simulink model "F16ASYM_Controlled_AoA"  (R2012b)
settings: Solver=ode3  SolverMode=SingleTasking  StartTime=0.0  StopTime=inf  FixedStep=T_sim  RelTol=1e-3
InitFcn:
  | load('NN_c_weights_Last_stable.mat')
values from neighbouring files (symbols this model uses):
  K_b_AoA = params(3)    [Cost_function.m]
  K_b_q = params(4)    [Cost_function.m]
  learning = 20    [Scheduling_desing.m]
  Model_used_flag = 1    [Scheduling_desing.m]
  reg_param = 0.5    [Scheduling_desing.m]
  T_sim = 0.02    [Scheduling_desing.m]
  tau_AoA = params(1)    [Cost_function.m]
  tau_q = params(2)    [Cost_function.m]
  Theta_1_roll_last = [0.00183613313267 0.00115998993235 0.0006676025148 0.00194921904952 0.00134963559861 0.00034352059664 0.000447169388141 0.00146749660935 0.00110199952389 7.77922383894e-05 0.00109492833348 0.00192687590535 ... (360 elements, 30x12)]    [NN_i_weights_LAST_STABLE.mat]
  Theta_2_roll_last = [0.000469743069697 0.000355923851088 0.00180035760697 0.00191855117771 0.00118851504447 0.0013331642065 0.0013164316578 0.000643981263341 0.00176817665434 0.000113802099363 0.000426534542462 0.00113815782354 ... (620 elements, 20x31)]    [NN_i_weights_LAST_STABLE.mat]
  Theta_3_roll_last = [9.62071520568e-05 -0.000389870886846 2.08260845013e-05 0.000140787743673 -0.000917525755397 -0.0014324207578 -0.00154701573815 -0.00131544476264 -0.00101205584381 5.06515794689e-05 -0.00111443483676 -0.00143957416141 ... (21 elements, 1x21)]    [NN_i_weights_LAST_STABLE.mat]
  V_long_lastA_w_z = [0.352826086601 -0.253633004548 -0.642535042878 0.237749930435 -0.618390629538 0.858074761295 0.268211230628 -0.448715080196 -0.0406384631192 0.401147605577 0.60598427709 0.0500551915851 ... (300 elements, 30x10)]    [NN_i_weights_LAST_STABLE.mat]
  V_long_lastAoA = [0.0774300162379 0.0911421319631 0.0352371192557 0.0542170286952 0.0651171200844 0.0177112012707 0.0982957728448 0.000259994642558 0.0194724569123 0.0466321328252 0.0556687953852 0.0252668067142 ... (300 elements, 30x10)]    [NN_i_weights_LAST_STABLE.mat]
  V_roll_last = [0.0540918675943 0.0557493347212 0.0839792276608 0.0460576391794 0.0671229058124 0.100220403067 0.0722493281881 0.0648875457457 0.00447599349201 0.0607299103823 0.0488037966361 0.0176785979393 ... (360 elements, 30x12)]    [NN_i_weights_LAST_STABLE.mat]
  V_yaw_last = [0.0965149149679 0.00833616709545 0.0365734360076 0.0523944217566 0.00790252078455 0.0700053845887 0.0345164868709 0.0111568465295 0.094060639546 0.0205483560006 0.000798047494256 0.0862769385758 ... (360 elements, 30x12)]    [NN_i_weights_LAST_STABLE.mat]
  velocity = M_eval_sche(I,J)*a    [Scheduling_desing.m]
  W_long_lastA_w_z = [-0.0522913429974 0.00385484301394 -0.00465489482472 -0.0139416219936 0.00295196421483 -0.013027768541 0.00585545058915 0.00278802233571 -0.00906272782329 -0.000396112031465 0.00405849743321 0.00509668457818 ... (31 elements, 1x31)]    [NN_i_weights_LAST_STABLE.mat]
  W_long_lastAoA = [-0.0192589013922 0.00873109909713 0.00432649597332 0.0420946902441 0.0293366820194 0.0351497798191 0.0234952374236 0.0360841187718 0.0112233388211 0.030147202199 0.0369533138617 0.00218839076415 ... (31 elements, 1x31)]    [NN_i_weights_LAST_STABLE.mat]
  W_roll_last = [-0.0006515532842 0.000535485585715 0.000550946920743 0.000806030945453 0.00045976209382 0.00065557954304 0.000945902185602 0.00070191398535 0.000635215543728 4.66501377412e-05 0.000597079583757 0.000485790566765 ... (31 elements, 1x31)]    [NN_i_weights_LAST_STABLE.mat]
  W_yaw_last = [-4.34263633305e-05 8.83823048922e-05 1.65575463724e-05 3.60293102233e-05 5.19752447623e-05 7.06399280852e-06 7.02425975821e-05 3.62680255076e-05 1.29996379937e-05 8.05072914397e-05 2.39941870661e-05 2.52427840574e-06 ... (31 elements, 1x31)]    [NN_i_weights_LAST_STABLE.mat]
undefined symbols (not defined in the file or in its folder): a1, alpha_map_eval, B, beta_map_eval, C_L_0, DiscIntNeverNeededParam, fi_flag_Simulink, G_eval, H_sq, H_sq_autotrim, k_B, m_B, M_sq, M_sq_autotrim, sigbuilder_block, Stall_curve, trim_control, trim_state, trim_throttle, V_Comp_A_w_z_last, V_Comp_last, V_roll_lastMOD, W_Comp_A_w_z_last, W_Comp_last, W_roll_lastMOD
libraries: Adaptive_FaultTolerantControl x43, dspsigops x29, F16_Actuator_Library x14, simulink x8, aerolibatmos2 x7, dsparch4 x6, simulink_extras x5, aerolibtransform2 x5, qcatlib x4, dspmtrx3 x3, dspvision x2, dspsnks4 x2
(part 3 of 11)

== system F16ASYM_Controlled_AoA/F-16 Non-linear Plant/SYM and ASYM model: RECONFIGURABLE ==
  note: Add the sytmetric
      |  deflection of the LEFs
  note: OUTPUTS
      | States:
      | 1. DEV North Position
      | 2. DEV East position
      | 3. DEV Altitude
      | 4.DEV  Phi
      | 5. DEV Theta
      | 6. DEV Psi
      | 7. DEV Total velocity
      | 8.DEV alpha in rad
      | 9.DEV  beta in rads
      | 10. DEV P
      | 11. DEV Q
      | 12. DEV R
      | 13. DEV POW
      |
      | Other outputs:
      | Accels of CG:
      | 14. anx_cg
      | 15. any_cg
      | 16. anz_cg
      | 17. mach
      | 18. qbar
      | 19. ps   Static Pressure
  note: Fidelity Flage tells nlplant
      | which Model to use:
      | 0: Low Fidelity
      | 1: High Fidelity
  note: INPUTS
      | States:
      | 1. North Position
      | 2. East position
      | 3. Altitude
      | 4. Phi
      | 5. Theta
      | 6. Psi
      | 7. Total velocity
      | 8. alpha in rad
      | 9. beta in rads
      | 10. P
      | 11. Q
      | 12. R
      | 13. POW
      |
      | Controls:
      |
      | 14. Throttle
      | 15. Elevator_L in deg
      | 16. Elevator_R in deg
      | 17. Aileron_L
      | 18. Aileron_R
      | 19. Rudder
      | 20. LEF_L
      | 21. LEF_R
      |
      | 22. Fidelity Flag
      |
      | 23. Model used: Asymetric or Symetric
      |
      | RECONFIGURATION PARAMETERS
      |
      | 24. mass  Estimated mass
      | 25. S_current_L
      | 26. S_current_R
      | 27. S_fin_current
      | 28. x_cg
      | 29. Jy
      | 30. Jxz
      | 31. Jz
      | 32. Jx
      | 33. EFF_el_L
      | 34. EFF_el_R
      | 35. EFF_ail_L
      | 36. EFF_ail_R
      | 37. EFF_rud
      | 38. EFF_lef_L
      | 39. EFF_lef_R
      | 40. Delta_C_Lift_X
      | 41. Delta_C_Drag_X
      | 42. Delta_C_m_X
  note: Mdoel used  Flage tells the plant
      |  if Asymetric or symetric model is used:
      | 0: Symetric Model
      | 1: Asymetric model
  States : Inport
  Reconf params : Inport  Port=2
  Control Comands : Inport  Port=3
  Acels actual : Scope
      settings: YMin=-0.04  YMax=0.09  SaveName=ScopeData14
  Actuators Dynamcis : Subsystem  TreatAsAtomicUnit=on
  Bus Creator : BusCreator  Inputs=12
  Bus Creator1 : BusCreator  Inputs=2
  Bus Selector : BusSelector  OutputSignals=Blockades,Blockade now,Reconfig signal
  Demux : Demux  Outputs=[13 6]
  Demux1 : Demux  Outputs=8
  F16 nlsim nlplant Asymetrical : MATLABFcn  MATLABFcn=nlplantASYM_Reconf  OutputDimensions=19  OutputSignalType=real
  Fidelity Flag : Constant  Value=fi_flag_Simulink
  Integrate F16 State Derivatives : Integrator  InitialCondition=trim_state
  Leading Edge Flap:Symetric deflection : Subsystem
  Model used flag : Constant  Value=Model_used_flag
  Mux1 : Mux  Inputs=8
  Mux2 : Mux  Inputs=[23 19]
  Mux5 : Mux  Inputs=[13 8 1 1]
  Rotation Angles to Direction Cosine Matrix : aerolibtransform2/Rotation Angles to Direction Cosine Matrix  rotationOrder=ZYX
  Selector : Selector  InputPortWidth=13  IndexOptions=Index vector (dialog)  Indices=[1:3]  OutputSizes=1
  Selector1 : Selector  InputPortWidth=13  IndexOptions=Index vector (dialog)  Indices=[1:3]  OutputSizes=1
  Selector2 : Selector  InputPortWidth=13  IndexOptions=Index vector (dialog)  Indices=[7]  OutputSizes=1
  Selector3 : Selector  InputPortWidth=13  IndexOptions=Index vector (dialog)  Indices=[8:9]  OutputSizes=1
  Selector4 : Selector  InputPortWidth=13  IndexOptions=Index vector (dialog)  Indices=[10:12]  OutputSizes=1
  Selector5 : Selector  InputPortWidth=13  IndexOptions=Index vector (dialog)  Indices=[4:6]  OutputSizes=1
  Selector6 : Selector  InputPortWidth=6  IndexOptions=Index vector (dialog)  Indices=[1:3]  OutputSizes=1
  Selector7 : Selector  InputPortWidth=3  IndexOptions=Index vector (dialog)  Indices=[3 2 1]  OutputSizes=1
  Selector9 : Selector  InputPortWidth=13  IndexOptions=Index vector (dialog)  Indices=[10:12]  OutputSizes=1
  Signal Specification : SignalSpecification  Dimensions=19
  Sum1 : Sum  Inputs=|++  SaturateOnIntegerOverflow=on  InputSameDT=on  OutDataTypeStr=Inherit: Same as first input
  Sum9 : Sum  Inputs=|++  SaturateOnIntegerOverflow=on  InputSameDT=on  OutDataTypeStr=Inherit: Same as first input
  Output_bus : Outport
  Actual control def : Outport  Port=2
  wires:
  Integrate F16 State Derivatives/1 -> Selector5/1, Selector4/1, Selector3/1, Selector2/1, Selector/1, Bus Creator/2  "States_out"
  Rotation Angles to Direction Cosine Matrix/1 -> Bus Creator/10  "DCM_b"
  Bus Creator/1 -> Output_bus/1, Leading Edge Flap:Symetric deflection/1(state)
  Fidelity Flag/1 -> Mux5/3
  Control Comands/1 -> Demux1/1
  States/1 -> Mux5/1
  Mux2/1 -> F16 nlsim nlplant Asymetrical/1  "INPUTS"
  F16 nlsim nlplant Asymetrical/1 -> Demux/1  "OUTPUTS"
  Actuators Dynamcis/2(Dec_Control_def) -> Mux5/2
  Model used flag/1 -> Mux5/4
  Demux1/8 -> Sum1/1
  Demux1/7 -> Sum9/1
  Leading Edge Flap:Symetric deflection/1(delta_lef (deg)) -> Bus Creator1/1, Sum1/2, Sum9/2  "Symetric_LEF_defl"
  Demux1/5 -> Mux1/5
  Demux1/3 -> Mux1/3
  Demux1/1 -> Mux1/1
  Demux1/2 -> Mux1/2
  Demux1/4 -> Mux1/4
  Demux1/6 -> Mux1/6
  Sum9/1 -> Mux1/7
  Sum1/1 -> Mux1/8
  Mux1/1 -> Actuators Dynamcis/1(Control_commands)
  Selector9/1 -> Acels actual/1
  Actuators Dynamcis/3(Throttle_meas) -> Bus Creator/12  "Throttle"
  Demux/1 -> Selector9/1, Bus Creator/1, Selector1/1, Integrate F16 State Derivatives/1  "States_dot_out"
  Selector/1 -> Bus Creator/4  "X_e"
  Selector1/1 -> Bus Creator/5  "V_e"
  Selector2/1 -> Bus Creator/6  "TAS"
  Selector3/1 -> Bus Creator/7  "alpha ; beta"
  Selector4/1 -> Bus Creator/8  "p;q;r"
  Selector5/1 -> Selector7/1, Bus Creator/9  "euler"
  Selector6/1 -> Bus Creator/11  "an_b_CG"
  Demux/2 -> Selector6/1, Bus Creator/3  "Other outs"
  Selector7/1 -> Rotation Angles to Direction Cosine Matrix/1
  Mux5/1 -> Mux2/1  "INPUTS"
  Signal Specification/1 -> Actuators Dynamcis/4(Reconfig signal), Mux2/2
  Reconf params/1 -> Bus Selector/1
  Bus Selector/3 -> Signal Specification/1  "<Reconfig signal>"
  Bus Selector/1 -> Actuators Dynamcis/2(Blockades)  "<Blockades>"
  Bus Selector/2 -> Actuators Dynamcis/3(Blockade now)  "<Blockade now>"
  Bus Creator1/1 -> Actual control def/1
  Actuators Dynamcis/1(Control Defl Plot) -> Bus Creator1/2  "actual_control_defl"

== system F16ASYM_Controlled_AoA/NDI/NDI: NO RECONFIG ==
  note: These two block MUST be evaluated at the same dynamics X
      | and control deflections delta*
      |
      |
      | delta* are a given set of control deflection: can be either the initial trim set
      | or the previous deflections
  Est reconf : Inport
  Angular_acc_des (rad/s^2) : Inport  Port=2
  All_meas : Inport  Port=3
  Control_defl for eval : Inport  Port=4
  Bus Selector : BusSelector  OutputSignals=signal1.omega_b meas (rad/s),signal2.q (Pa),signal1.Alt meas (m),signal1.V_TAS (m/s),signal1.AoA meas (rad),signal1.SS meas (rad),signal1.Throttle_meas
  Demux : Demux  Outputs=3
  Dim_less : Subsystem
  Inversion : Sum  Inputs=|+-
  Memory : Memory  X0=[0,0,0]
  Mom Coefficients gradient with control deflections at the given dynamics X: It performs perturbations theory arroun the given control deflections : MATLABFcn  MATLABFcn=Moms_Coeff_Grad_estimator  OutputDimensions=21  OutputSignalType=real
  Mux : Mux  Inputs=3
  Mux1 : Mux  Inputs=7
  Pre-Inverter : MATLAB Function  TreatAsAtomicUnit=on
  Reshape : Reshape  OutputDimensionality=Customize  OutputDimensions=[k_B,m_B]
  Terminator : Terminator
  Trim controls Asym In LEFs: Additionaly from dLEF : Constant  Commented=on  Value=[trim_control(1),trim_control(1),trim_control(2),-trim_control(2),trim_control(3),0,0]
  "f(x)  Mom Coefficients due to the dynamics: Coefficients model with control inputs " : MATLABFcn  MATLABFcn=Moms_Coeff_estimator  OutputDimensions=3  OutputSignalType=real
  Virtual Control Commands : Outport
  B online : Outport  Port=2
  Control_defl evald : Outport  Port=3
  Mom coef comm : Outport  Port=4
  wires:
  Est reconf/1 -> Terminator/1
  Reshape/1 -> B online/1
  Mom Coefficients gradient with control deflections at the given dynamics X: It performs perturbations theory arroun the given control deflections/1 -> Reshape/1
  Mux/1 -> Memory/1, Inversion/1
  Bus Selector/7 -> Mux1/6  "<Throttle_meas>"
  Mux1/1 -> Mom Coefficients gradient with control deflections at the given dynamics X: It performs perturbations theory arroun the given control deflections/1, "f(x)  Mom Coefficients due to the dynamics: Coefficients model with control inputs "/1
  Control_defl for eval/1 -> Mux1/7, Control_defl evald/1
  Bus Selector/6 -> Mux1/4  "<SS meas (rad)>"
  Bus Selector/5 -> Mux1/3  "<AoA meas (rad)>"
  Bus Selector/4 -> Mux1/2  "<V_TAS (m/s)>"
  Bus Selector/3 -> Mux1/1  "<Alt meas (m)>"
  "f(x)  Mom Coefficients due to the dynamics: Coefficients model with control inputs "/1 -> Inversion/2  "f(x) or C_x"
  Dim_less/3(C_N des) -> Mux/3
  Dim_less/2(C_M des) -> Mux/2
  Dim_less/1(C_L des) -> Mux/1
  Pre-Inverter/3(N_comm) -> Dim_less/3(N_comm)
  Pre-Inverter/2(M_comm) -> Dim_less/2(M_comm)
  Pre-Inverter/1(L_comm) -> Dim_less/1(L_comm)
  Bus Selector/2 -> Dim_less/4(q)  "<q (Pa)>"
  All_meas/1 -> Bus Selector/1
  Demux/1 -> Pre-Inverter/1(p_dot_comm)
  Demux/3 -> Pre-Inverter/3(r_dot_comm)
  Demux/2 -> Pre-Inverter/2(q_dot_comm)
  Angular_acc_des (rad/s^2)/1 -> Demux/1
  Bus Selector/1 -> Mux1/5, Pre-Inverter/4(omega_b)  "<omega_b meas (rad/s)>"
  Inversion/1 -> Virtual Control Commands/1
  Memory/1 -> Mom coef comm/1

== system F16ASYM_Controlled_AoA/NDI/NDI: RECONFIG ==
  note: These two block MUST be evaluated at the same dynamics X
      | and control deflections delta*
      |
      |
      | delta* are a given set of control deflection: can be either the initial trim set
      | or the previous deflections
  note: INPUTS
      | States:
      |
      | 1. Altitude
      | 2. TAS velocity
      | 3. alpha in rad
      | 4. beta in rads
      | 5. P
      | 6. Q
      | 7. R
      | 8. Throttle
      | 9. Elevator_L in deg
      | 10. Elevator_R in deg
      | 11. Aileron_L
      | 12. Aileron_R
      | 13. Rudder
      | 14. LEF_L
      | 15. LEF_R
      |
      | RECONFIGURATION PARAMETERS
      |
      | 16. mass  Estimated mass
      | 17. S_current_L
      | 18. S_current_R
      | 19. S_fin_current
      | 20. x_cg
      | 21. Jy
      | 22. Jxz
      | 23. Jz
      | 24. Jx
      | 25. EFF_el_L
      | 26. EFF_el_R
      | 27. EFF_ail_L
      | 28 EFF_ail_R
      | 29. EFF_rud
      | 30. EFF_lef_L
      | 31. EFF_lef_R
      | 32. Delta_C_Lift_X
      | 33. Delta_C_Drag_X
      | 34. Delta_C_m_X
  Est reconf : Inport
  Angular_acc_des (rad/s^2) : Inport  Port=2
  All_meas : Inport  Port=3
  Control_defl for eval : Inport  Port=4
  Bus Selector : BusSelector  OutputSignals=signal1.omega_b meas (rad/s),signal2.q (Pa),signal1.Alt meas (m),signal1.V_TAS (m/s),signal1.AoA meas (rad),signal1.SS meas (rad),signal1.Throttle_meas
  Bus Selector1 : BusSelector  OutputSignals=Reconfig signal
  Controls : Scope
      settings: SaveName=ScopeData19
  Demux : Demux  Outputs=3
  Dim_less : Subsystem
  Inversion : Sum  Inputs=|+-
  Memory : Memory  X0=[0,0,0]
  Mom Coefficients gradient with control deflections at the given dynamics X: It performs perturbations theory arroun the given control deflections : MATLABFcn  MATLABFcn=Moms_Coeff_Grad_Reconf_estimator  OutputDimensions=21  OutputSignalType=real
  Mux : Mux  Inputs=3
  Mux1 : Mux  Inputs=7
  Mux2 : Mux  Inputs=[15 19]
  Plant : Scope
      settings: SaveName=ScopeData11
  Pre-Inverter : MATLAB Function  TreatAsAtomicUnit=on
  Reshape : Reshape  OutputDimensionality=Customize  OutputDimensions=[k_B,m_B]
  Signal Specification : SignalSpecification  Dimensions=19
  Trim controls Asym In LEFs: Additionaly from dLEF : Constant  Commented=on  Value=[trim_control(1),trim_control(1),trim_control(2),-trim_control(2),trim_control(3),0,0]
  f(x)  Mom Coefficients due to the dynamics: Coefficients model with control inputs : MATLABFcn  MATLABFcn=Moms_Coeff_Reconf_estimator  OutputDimensions=3  OutputSignalType=real
  Virtual Control Commands : Outport
  B online : Outport  Port=2
  Control_defl evald : Outport  Port=3
  Mom coef comm : Outport  Port=4
  wires:
  Inversion/1 -> Controls/1, Virtual Control Commands/1
  Bus Selector/1 -> Pre-Inverter/4(omega_b), Mux1/5  "<omega_b meas (rad/s)>"
  Angular_acc_des (rad/s^2)/1 -> Demux/1
  Demux/2 -> Pre-Inverter/2(q_dot_comm)
  Demux/3 -> Pre-Inverter/3(r_dot_comm)
  Demux/1 -> Pre-Inverter/1(p_dot_comm)
  All_meas/1 -> Bus Selector/1
  Bus Selector/2 -> Dim_less/4(q)  "<q (Pa)>"
  Pre-Inverter/1(L_comm) -> Dim_less/1(L_comm)
  Pre-Inverter/2(M_comm) -> Dim_less/2(M_comm)
  Pre-Inverter/3(N_comm) -> Dim_less/3(N_comm)
  Dim_less/1(C_L des) -> Mux/1
  Dim_less/2(C_M des) -> Mux/2
  Dim_less/3(C_N des) -> Mux/3
  f(x)  Mom Coefficients due to the dynamics: Coefficients model with control inputs/1 -> Plant/1, Inversion/2  "f(x) or C_x"
  Bus Selector/3 -> Mux1/1  "<Alt meas (m)>"
  Bus Selector/4 -> Mux1/2  "<V_TAS (m/s)>"
  Bus Selector/5 -> Mux1/3  "<AoA meas (rad)>"
  Bus Selector/6 -> Mux1/4  "<SS meas (rad)>"
  Control_defl for eval/1 -> Mux1/7, Control_defl evald/1
  Bus Selector/7 -> Mux1/6  "<Throttle_meas>"
  Mux/1 -> Inversion/1, Memory/1
  Mom Coefficients gradient with control deflections at the given dynamics X: It performs perturbations theory arroun the given control deflections/1 -> Reshape/1
  Reshape/1 -> B online/1
  Est reconf/1 -> Bus Selector1/1
  Bus Selector1/1 -> Signal Specification/1  "<Reconfig signal>"
  Mux1/1 -> Mux2/1
  Mux2/1 -> Mom Coefficients gradient with control deflections at the given dynamics X: It performs perturbations theory arroun the given control deflections/1, f(x)  Mom Coefficients due to the dynamics: Coefficients model with control inputs/1
  Signal Specification/1 -> Mux2/2
  Memory/1 -> Mom coef comm/1

== system F16ASYM_Controlled_AoA/P controller + adaptive Crossed NN + AWU+Lim+scheduling   in AoA/Body Rates Controller ==
  p_ref : Inport
  q_ref : Inport  Port=2
  r_ref : Inport  Port=3
  All_meas : Inport  Port=4
  Bus Creator : BusCreator
  Bus Creator1 : BusCreator
  Bus Creator2 : BusCreator
  Bus Selector : BusSelector  OutputSignals=signal1.omega_b meas (rad/s)
  Display1 : Display
  Mux : Mux  Inputs=3
  Ref Model and P Controller p : Adaptive_FaultTolerantControl/Ref Model and P Controller  tau=0.1  y_i=trim_state(10)  K_f=1  K_b=7
  Ref Model and P Controller q : Subsystem
  Ref Model and P Controller r : Adaptive_FaultTolerantControl/Ref Model and P Controller  tau=0.2  y_i=trim_state(12)  K_f=1  K_b=4
  Selector : Selector  InputPortWidth=3  IndexOptions=Index vector (dialog)  Indices=1  OutputSizes=1
  Selector1 : Selector  InputPortWidth=3  IndexOptions=Index vector (dialog)  Indices=2  OutputSizes=1
  Selector2 : Selector  InputPortWidth=3  IndexOptions=Index vector (dialog)  Indices=3  OutputSizes=1
  Sum : Sum  Inputs=+-|
  Sum1 : Sum  Inputs=+-|
  Sum2 : Sum  Inputs=+-|
  q_chanel vars : Outport
  p_chanel vars : Outport  Port=2
  r_chanel vars : Outport  Port=3
  Angular acc des (rad/s^2) : Outport  Port=4
  wires:
  All_meas/1 -> Bus Selector/1
  Bus Selector/1 -> Selector/1, Selector1/1, Selector2/1  "<omega_b meas (rad/s)>"
  p_ref/1 -> Ref Model and P Controller p/1
  Selector/1 -> Ref Model and P Controller p/2
  Ref Model and P Controller p/1 -> Mux/1
  Mux/1 -> Angular acc des (rad/s^2)/1
  q_ref/1 -> Ref Model and P Controller q/1(y_ref)
  Selector1/1 -> Ref Model and P Controller q/2(y_meas)
  r_ref/1 -> Ref Model and P Controller r/1
  Ref Model and P Controller q/1(y_des_dot) -> Mux/2
  Ref Model and P Controller r/1 -> Mux/3
  Ref Model and P Controller p/2 -> Bus Creator/1  "p_sf_dot"
  Ref Model and P Controller p/3 -> Sum/1, Bus Creator/2  "p_sf"
  Sum/1 -> Display1/1, Bus Creator/3  "p_err"
  Bus Creator/1 -> p_chanel vars/1
  Bus Creator1/1 -> q_chanel vars/1
  Bus Creator2/1 -> r_chanel vars/1
  Selector2/1 -> Ref Model and P Controller r/2
  Ref Model and P Controller p/4 -> Sum/2
  Ref Model and P Controller p/5 -> Bus Creator/4  "K_b_p"
  Ref Model and P Controller q/2(y_c_ff_dot) -> Bus Creator1/1  "q_sf_dot"
  Ref Model and P Controller q/3(y_c) -> Sum1/1, Bus Creator1/2  "q_sf"
  Sum1/1 -> Bus Creator1/3  "q_err"
  Ref Model and P Controller q/4(y_meas_out) -> Sum1/2
  Ref Model and P Controller q/5(k_b param) -> Bus Creator1/4  "K_b_q"
  Ref Model and P Controller r/2 -> Bus Creator2/1  "r_sf_dot"
  Ref Model and P Controller r/3 -> Sum2/1, Bus Creator2/2  "r_sf"
  Sum2/1 -> Bus Creator2/3  "r_err"
  Ref Model and P Controller r/4 -> Sum2/2
  Ref Model and P Controller r/5 -> Bus Creator2/4  "K_b_r"

== matlab function F16ASYM_Controlled_AoA/Primary Controller/P controller + adaptive Crossed NN + AWU+Lim /Physical limitation/max deflections estimator ==
  data: v_comm input; max_defl output; B parameter
function max_defl = Max_defl(v_comm,B)
sup_limit = [24,24,21,21,29,25,25];
inf_limit = [-24,-24,-21,-21,-29,0,0];

def=B;
for i=1:3
    def(i,:) = B(i,:).*sign(v_comm(i));
end
def_avg = mean(def,1);

max_defl = zeros(7,1);
for i=1:7
    if def_avg(1,i)>0
        max_defl(i) = sup_limit(i);
    else
        max_defl(i) = inf_limit(i);
    end
end

== matlab function F16ASYM_Controlled_AoA/Control allocator/Control allocator: NO RECONF/MATLAB Function ==
  data: Deflections input; Saturations output; Sup_lim input; Inf_lim input
function Saturations = Saturations(Deflections,Sup_lim,Inf_lim)
Saturations=zeros(7,1);

for i=1:7
    
    if Deflections(i)>=Sup_lim(i)
        Saturations(i)=1;
    elseif Deflections(i)<=Inf_lim(i)
        Saturations(i)=-1;
    else
        Saturations(i)=0;
    end
end

== matlab function F16ASYM_Controlled_AoA/Anti-windup Calculation/Anti-windup: NO reconfigurable/Ang Accel ==
  data: L input; p_dot output; q_dot output; r_dot output; M input; N input; omega_b input
function [p_dot,q_dot,r_dot] = Ang_accel(L,M,N,omega_b)
Jy  = 75673.6;
Jxz = 1331.4; 
Jz  = 85552.1;  
Jx  = 12874.8;
h_E = 216.9;

denom = Jx*Jz - Jxz*Jxz;

% % C1 = ((Jy - Jz)  * Jz  - (Jxz * Jxz))/ Gamma;
% % C2 = ((Jx - Jy + Jz ) * Jxz ) / Gamma;
% % C3 = Jz / Gamma;
% % C4 = Jxz / Gamma;
% % C5 = (Jz - Jx) / Jy;
% % C6 = Jxz / Jy ;
% % C7 = 1 / Jy;
% % C8 = (Jx * (Jx - Jy ) + Jxz * Jxz) / Gamma;
% % C9 = Jx / Gamma;


p_dot =  (Jz*L + Jxz*N - (Jz*(Jz-Jy)+Jxz*Jxz)*omega_b(2)*omega_b(3) + Jxz*(Jx-Jy+Jz)*omega_b(1)*omega_b(2) + Jxz*omega_b(2)*h_E)/denom;

q_dot = (M + (Jz-Jx)*omega_b(1)*omega_b(3) - Jxz*(omega_b(1)*omega_b(1)-omega_b(3)*omega_b(3)) - omega_b(3)*h_E)/Jy;


r_dot = (Jx*N + Jxz*L + (Jx*(Jx-Jy)+Jxz*Jxz)*omega_b(1)*omega_b(2) - Jxz*(Jx-Jy+Jz)*omega_b(2)*omega_b(3) +  Jx*omega_b(2)*h_E)/denom;

== matlab function F16ASYM_Controlled_AoA/Primary Controller/P controller + adaptive Crossed NN + AWU+Lim /Complete crossed On-line (adaptive) multi-layer NN/Complete crossed On-line (adaptive) multi-layer NN: AoA/Cross NN ==
  data: X_bar input size=[25,1]; v_ad_comp output; e input; K_roll input; Ks_long input; Ks_yaw input; B input; Learnign_rate input size=1; Reg_param input size=1; AWU input; W input size=[3,51]; V input size=[50,25]; v_ad output; Z_norm_unit output; T_sim parameter; W_update output; V_update output
function [v_ad_comp,v_ad,Z_norm_unit,W_update,V_update]  = Cross_NN(X_bar,e, K_roll,Ks_long,Ks_yaw,B,Learnign_rate,Reg_param,AWU,W,V,T_sim)

%% Compute prelimiary parametes
P_roll=1/K_roll;
P_long = [   1/Ks_long(1) , 1/(Ks_long(1)^2+Ks_long(1)*Ks_long(2));
     1/(Ks_long(1)^2+Ks_long(1)*Ks_long(2)) ,(Ks_long(1)^2+Ks_long(1)*Ks_long(2)+1)/(Ks_long(2)^2*Ks_long(1)+Ks_long(2)*Ks_long(1)^2) ];
P_yaw = [   1/Ks_yaw(1) , 1/(Ks_yaw(1)^2+Ks_yaw(1)*Ks_yaw(2));
     1/(Ks_yaw(1)^2+Ks_yaw(1)*Ks_yaw(2)) ,(Ks_yaw(1)^2+Ks_yaw(1)*Ks_yaw(2)+1)/(Ks_yaw(2)^2*Ks_yaw(1)+Ks_yaw(2)*Ks_yaw(1)^2) ];
 
 P = blkdiag(P_roll,P_long,P_yaw);



zeta= e'*P*B;
% Introduce Anti-windup
K_awu = 1.2;
zeta = zeta - K_awu*AWU'.*T_sim; 
% if norm(AWU)~=0
%     Learnign_rate=0;
% end
% Convergence limitation
if norm(zeta)>2/(T_sim*Learnign_rate*Reg_param)
    zeta = (zeta./norm(zeta)).*(1.8/(T_sim*Learnign_rate*Reg_param));
end
%% Feedforward
z = V*X_bar;
s=sigmoid(V*X_bar);

sigma = [1 ; s ];
% v_ad = W*sigma;

sigma_grad = (sigma.*(ones(size(sigma))-sigma));

%% Compute the gradients or adaptation laws
Gamma_w= Learnign_rate; % W learnign rate
Gamma_v= Learnign_rate; %V learning rate
lambda = Reg_param;

V_dot=zeros(size(V));
W_dot=zeros(size(W));

W_dot= -Gamma_w*(  (sigma - sigma_grad.*[1;z] )*zeta  )';
W_dot(:,2:end)= W_dot(:,2:end) - Gamma_w*lambda*norm(zeta)*(W(:,2:end));

M = W'*zeta'.*sigma_grad ;
V_dot= -Gamma_v*( M(2:end)*X_bar'  );
V_dot(:,2:end)= V_dot(:,2:end) - Gamma_v*lambda*norm(zeta).*V(:,2:end);


% % % % Other way: Based on notes of Andrew NG
% % % 
% % % delta2=W'*zeta'.*sigma_grad;
% % % 
% % % V_dot = - Gamma_v*( delta2(2:end)*X_bar');
% % % V_dot(:,2:end)= V_dot(:,2:end) - Gamma_v*lambda*norm(zeta).*V(:,2:end);
% % % 
% % % W_dot = - Gamma_w*( sigma*zeta)';
% % % W_dot(:,2:end)= W_dot(:,2:end) - Gamma_w*lambda*norm(zeta)*(W(:,2:end));



%% Adaptation
W_update = W + T_sim*W_dot;
V_update = V + T_sim*V_dot;

%% Re-compute v_ad

s=sigmoid(V_update*X_bar);

sigma = [1 ; s(:,1) ];
v_ad = W_update*sigma;

%% Compute v_ad_comp
Z = [ V,zeros(size(V,1),size(W,2));
    zeros(size(W,1),size(V,2)),W];
    
Z_norm = norm(Z,'fro');
Z_max = 2*min(size(W,1),size(W,2) )*min( size(V,1),size(V,2) );
Z_norm_unit = Z_norm;

K_r0= 0.02;
K_r1= 0;
v_r0 = -K_r0*zeta';
v_r1 = -K_r1*(Z_norm+Z_max)*zeta';

v_ad_comp = v_ad + v_r1 +v_r0;


end

== system F16ASYM_Controlled_AoA/P controller + adaptive Crossed NN + AWU+Lim+scheduling   in AoA/Complete crossed On-line (adaptive) multi-layer NN: AoA ==
  v_ad^ prev : Inport
  All_meas : Inport  Port=2
  NN variables : Inport  Port=3
  AWU : Inport  Port=4
  B : Constant  Value=[1 0 0;0 0 0;0 1 0;0 0 0;0 0 1]
  Bus Selector : BusSelector  OutputSignals=p_chanel_vars,Long chanel,beta_r_chanel
  Bus Selector1 : BusSelector  OutputSignals=p_err,p_sf,p_sf_dot,K_b_p
  Bus Selector2 : BusSelector  OutputSignals=signal1.Alt meas (m),signal2.Mach,signal1.AoA meas (rad),signal1.SS meas (rad),signal1.omega_b meas (rad/s)
  Bus Selector3 : BusSelector  OutputSignals=alpha_chanel vars.alpha_err,q_chanel_vars.q_err,alpha_chanel vars.alpha_sf,alpha_chanel vars.alpha_sf_dot,q_chanel_vars.q_sf_dot,alpha_chanel vars.K_b_alpha,q_chanel_vars.K_b_q
  Bus Selector4 : BusSelector  OutputSignals=beta_chanel vars.beta_err,r_chanel vars.r_err,beta_chanel vars.beta_sf,beta_chanel vars.beta_sf_dot,r_chanel vars.r_sf_dot,beta_chanel vars.K_b_beta,r_chanel vars.K_b_r
  C Learning rate : Constant  Value=learning  SampleTime=T_sim
  C Reg param : Constant  Value=reg_param  SampleTime=T_sim
  Constant : Constant
  Cross NN : MATLAB Function  TreatAsAtomicUnit=on
  Display : Display
  Divide : Product  Inputs=**
  Divide1 : Product  Inputs=**
  Memory2 : Memory  X0=V_Comp_last
  Memory3 : Memory  X0=W_Comp_last
  Mux1 : Mux  Inputs=9
  Mux10 : Mux  Inputs=3
  Mux2 : Mux  Inputs=3
  Mux{3..4,6..7} (4 alike) : Mux  Inputs=2
  Mux5 : Mux  Inputs=5
  Mux8 : Mux  Inputs=5
  Mux9 : Mux  Inputs=[9 3 5 5 3]
  Scope : Scope
      settings: SaveName=ScopeData8
  Selector : Selector  InputPortWidth=3  IndexOptions=Index vector (dialog)  Indices=1  OutputSizes=1
  Selector1 : Selector  InputPortWidth=3  IndexOptions=Index vector (dialog)  Indices=3  OutputSizes=1
  Terminator : Terminator
  Terminator1 : Terminator
  To Workspace : ToWorkspace  VariableName=V_Comp_last  SampleTime=-1
      settings: MaxDataPoints=1
  To Workspace1 : ToWorkspace  VariableName=W_Comp_last  SampleTime=-1
      settings: MaxDataPoints=1
  dem-less : Gain  Gain=T_sim
  dem-less1 : Gain  Gain=T_sim
  dem-less2 : Gain  Gain=T_sim^2
  dem-less3 : Gain  Gain=T_sim
  dem-less4 : Gain  Gain=T_sim^2
  dim-less : Gain  Gain=1/15000
  v_ad^ : Outport
  wires:
  Bus Selector/3 -> Bus Selector4/1  "<beta_r_chanel>"
  Bus Selector/2 -> Bus Selector3/1  "<Long chanel>"
  Bus Selector/1 -> Bus Selector1/1  "<p_chanel_vars>"
  NN variables/1 -> Bus Selector/1
  Bus Selector2/5 -> Selector1/1, Selector/1  "<omega_b meas (rad/s)>"
  dim-less/1 -> Mux1/2
  Divide1/1 -> Mux1/6
  Divide/1 -> Mux1/4
  Bus Selector2/1 -> dim-less/1  "<Alt meas (m)>"
  All_meas/1 -> Bus Selector2/1
  Constant/1 -> Mux1/1
  Bus Selector1/3 -> dem-less/1  "<p_sf_dot>"
  Selector/1 -> Mux1/8
  Bus Selector2/4 -> Mux1/7  "<SS meas (rad)>"
  Bus Selector2/2 -> Divide/2, Mux1/3, Divide/1  "<Mach>"
  Bus Selector2/3 -> Divide1/1, Mux1/5, Divide1/2  "<AoA meas (rad)>"
  Bus Selector1/4 -> [K_roll]  "<K_b_p>"
  Bus Selector1/2 -> Mux2/2  "<p_sf>"
  Bus Selector1/1 -> [e_roll], Mux2/1  "<p_err>"
  dem-less/1 -> Mux2/3
  dem-less2/1 -> Mux5/5
  dem-less1/1 -> Mux5/4
  Mux4/1 -> [Ks_long]
  Bus Selector3/6 -> Mux4/1  "<K_b_alpha>"
  Bus Selector3/7 -> Mux4/2  "<K_b_q>"
  Bus Selector3/5 -> dem-less2/1  "<q_sf_dot>"
  Bus Selector3/4 -> dem-less1/1  "<alpha_sf_dot>"
  Bus Selector3/1 -> Mux5/1, Mux3/1  "<alpha_err>"
  Bus Selector3/2 -> Mux5/2, Mux3/2  "<q_err>"
  Bus Selector3/3 -> Mux5/3  "<alpha_sf>"
  Mux3/1 -> [e_long]  "e"
  dem-less3/1 -> Mux8/4
  Bus Selector4/3 -> Mux8/3  "<beta_sf>"
  Bus Selector4/4 -> dem-less3/1  "<beta_sf_dot>"
  Bus Selector4/5 -> dem-less4/1  "<r_sf_dot>"
  Bus Selector4/7 -> Mux6/2  "<K_b_r>"
  Bus Selector4/6 -> Mux6/1  "<K_b_beta>"
  Mux6/1 -> [Ks_yaw]
  Bus Selector4/1 -> Mux8/1, Mux7/1  "<beta_err>"
  Bus Selector4/2 -> Mux8/2, Mux7/2  "<r_err>"
  Mux7/1 -> [e_yaw]  "e"
  dem-less4/1 -> Mux8/5
  Mux1/1 -> Mux9/1
  Mux2/1 -> Mux9/2
  Mux5/1 -> Mux9/3
  Mux8/1 -> Mux9/4
  v_ad^ prev/1 -> Mux9/5
  Mux9/1 -> Scope/1, Display/1, Cross NN/1(X_bar)
  Cross NN/3(Z_norm_unit) -> Terminator1/1
  C Reg param/1 -> Cross NN/8(Reg_param)
  C Learning rate/1 -> Cross NN/7(Learnign_rate)
  Cross NN/1(v_ad_comp) -> v_ad^/1
  Memory2/1 -> Cross NN/11(V)
  Memory3/1 -> Cross NN/10(W)
  B/1 -> Cross NN/6(B)
  Cross NN/2(v_ad) -> Terminator/1
  Cross NN/5(V_update) -> To Workspace/1, Memory2/1
  Cross NN/4(W_update) -> Memory3/1, To Workspace1/1
  Mux10/1 -> Cross NN/2(e)
  [e_roll] -> Mux10/1
  [e_long] -> Mux10/2
  [e_yaw] -> Mux10/3
  [K_roll] -> Cross NN/3(K_roll)
  [Ks_long] -> Cross NN/4(Ks_long)
  [Ks_yaw] -> Cross NN/5(Ks_yaw)
  Selector1/1 -> Mux1/9
  AWU/1 -> Cross NN/9(AWU)

== system F16ASYM_Controlled_AoA/P controller + adaptive Crossed NN + AWU+Lim+scheduling   in AoA/Lat_dir Dyn Inversion: beta_dot->r_c ==
  beta_dot_c : Inport
  All_meas : Inport  Port=2
  A_w_y : Selector  InputPortWidth=3  IndexOptions=Index vector (dialog)  Indices=2  OutputSizes=1
  Bus Selector : BusSelector  OutputSignals=signal1.AoA meas (rad),signal1.omega_b meas (rad/s),signal1.V_TAS (m/s),signal2.A_w_CG
  Divide1 : Product  Inputs=**
  Divide3 : Product  Inputs=**
  Divide4 : Product  Inputs=/*
  Divide5 : Product  Inputs=*/
  Selector : Selector  InputPortWidth=3  IndexOptions=Index vector (dialog)  Indices=1  OutputSizes=1
  Trigonometric Function : Trigonometry  Operator=cos
  Trigonometric Function3 : Trigonometry  Operator=tan
  "q_c " : Sum  Inputs=-++
  r_c : Outport
  wires:
  "q_c "/1 -> r_c/1
  Bus Selector/1 -> Trigonometric Function/1, Trigonometric Function3/1  "<AoA meas (rad)>"
  Bus Selector/2 -> Selector/1  "<omega_b meas (rad/s)>"
  Divide1/1 -> "q_c "/2
  Divide3/1 -> Divide4/1
  A_w_y/1 -> Divide4/2
  All_meas/1 -> Bus Selector/1
  Bus Selector/4 -> A_w_y/1  "<A_w_CG>"
  Divide4/1 -> "q_c "/3
  Bus Selector/3 -> Divide3/2  "<V_TAS (m/s)>"
  Trigonometric Function/1 -> Divide3/1, Divide5/2
  Divide5/1 -> "q_c "/1
  beta_dot_c/1 -> Divide5/1
  Trigonometric Function3/1 -> Divide1/1
  Selector/1 -> Divide1/2

== system F16ASYM_Controlled_AoA/P controller + adaptive Crossed NN + AWU+Lim+scheduling   in AoA/Long Dyn Inversion: alpha_dot ->q ==
  alpha_dot_c : Inport
  All_meas : Inport  Port=2
  Completed : Subsystem
  Manual Switch : ManualSwitch
  Simplified : Subsystem
  q_c : Outport
  wires:
  alpha_dot_c/1 -> Simplified/1(alpha_dot_c), Completed/1(alpha_dot_c)
  All_meas/1 -> Simplified/2(All_meas), Completed/2(All_meas)
  Completed/1(q_c) -> Manual Switch/1
  Simplified/1(q_c) -> Manual Switch/2
  Manual Switch/1 -> q_c/1

== system F16ASYM_Controlled_AoA/P controller + adaptive Crossed NN + AWU+Lim+scheduling   in AoA/Longitudinal controller in AoA ==
  A_w_z des : Inport
  AoA des (rad) : Inport  Port=2
  Anti-windup A_w_z : Inport  Port=3
  Anti-windup AoA : Inport  Port=4
  All meas : Inport  Port=5
  Bus Creator : BusCreator
  Bus Selector : BusSelector  OutputSignals=signal1.AoA meas (rad)
  Ref Model and P Controller : Subsystem
  Sum : Sum  Inputs=+-|
  Terminator : Terminator
  Terminator1 : Terminator
  Terminator2 : Terminator
  alpha_chanel vars : Outport
  alpha_dot_c : Outport  Port=2
  wires:
  All meas/1 -> Bus Selector/1
  Ref Model and P Controller/1(y_des_dot) -> alpha_dot_c/1
  Bus Selector/1 -> Ref Model and P Controller/2(y_meas)  "<AoA meas (rad)>"
  AoA des (rad)/1 -> Ref Model and P Controller/1(y_ref)
  A_w_z des/1 -> Terminator/1
  Anti-windup A_w_z/1 -> Terminator1/1
  Anti-windup AoA/1 -> Terminator2/1
  Ref Model and P Controller/2(y_c_ff_dot) -> Bus Creator/1  "alpha_sf_dot"
  Ref Model and P Controller/3(y_c) -> Sum/1, Bus Creator/2  "alpha_sf"
  Sum/1 -> Bus Creator/3  "alpha_err"
  Bus Creator/1 -> alpha_chanel vars/1
  Ref Model and P Controller/4(y_meas_out) -> Sum/2
  Ref Model and P Controller/5(k_b param) -> Bus Creator/4  "K_b_alpha"

== system F16ASYM_Controlled_AoA/P controller + adaptive Crossed NN + AWU+Lim+scheduling   in AoA/Physical limitation ==
  note: Converto to Angular accelerations
  v comm : Inport
  all meas : Inport  Port=2
  Ang Accel : MATLAB Function
  Bus Selector : BusSelector  OutputSignals=signal1.Alt meas (m),signal1.V_TAS (m/s),signal1.AoA meas (rad),signal1.SS meas (rad),signal1.omega_b meas (rad/s),signal1.Throttle_meas
  Bus Selector1 : BusSelector  OutputSignals=signal2.q (Pa),signal1.omega_b meas (rad/s)
  Demux : Demux  Outputs=3
  Display : Display
  Display1 : Display
  Display2 : Display
  Divide : Product  Inputs=**
  Divide1 : Product  Inputs=**
  Gain : Gain  Gain=-1
  Gain1 : Gain
  Mom coefficients that was reached : MATLABFcn  MATLABFcn=Moms_Coeff_estimator  OutputDimensions=3  OutputSignalType=real
  Moments : Subsystem
  Mux : Mux  Inputs=3
  Mux1 : Mux  Inputs=7
  Saturation Dynamic : simulink/Discontinuities/Saturation Dynamic  OutMin=[]  OutMax=[]  OutDataTypeStr=Inherit: Same as second input  OutDataType=fixdt(1, 16)  OutScaling=2^-10  DoSatur=off
  Sign : Signum
  Sign1 : Signum
  max deflections estimator : MATLAB Function  TreatAsAtomicUnit=on
  v limted : Outport
  wires:
  max deflections estimator/1(max_defl) -> Mux1/7
  Mux1/1 -> Mom coefficients that was reached/1
  Bus Selector/5 -> Mux1/5  "<omega_b meas (rad/s)>"
  Bus Selector/1 -> Mux1/1  "<Alt meas (m)>"
  Bus Selector/2 -> Mux1/2  "<V_TAS (m/s)>"
  Bus Selector/3 -> Mux1/3  "<AoA meas (rad)>"
  Bus Selector/4 -> Mux1/4  "<SS meas (rad)>"
  Bus Selector/6 -> Mux1/6  "<Throttle_meas>"
  Ang Accel/2(q_dot) -> Mux/2
  Ang Accel/3(r_dot) -> Mux/3
  Ang Accel/1(p_dot) -> Mux/1
  Bus Selector1/2 -> Ang Accel/4(omega_b)  "<omega_b meas (rad/s)>"
  Moments/3(N) -> Ang Accel/3(N)
  Moments/2(M) -> Ang Accel/2(M)
  Moments/1(L) -> Ang Accel/1(L)
  Bus Selector1/1 -> Moments/4(q)  "<q (Pa)>"
  Demux/3 -> Moments/3(C_N)
  Demux/2 -> Moments/2(C_M)
  Demux/1 -> Moments/1(C_L)
  Mom coefficients that was reached/1 -> Demux/1
  all meas/1 -> Bus Selector/1, Bus Selector1/1
  Mux/1 -> Gain1/1
  v comm/1 -> Saturation Dynamic/2, Display1/1, max deflections estimator/1(v_comm)
  Saturation Dynamic/1 -> Display/1, v limted/1
  Sign/1 -> Divide/1
  Gain1/1 -> Divide/2, Divide1/1, Sign1/1, Display2/1, Sign/1
  Sign1/1 -> Gain/1
  Divide/1 -> Saturation Dynamic/1
  Gain/1 -> Divide1/2
  Divide1/1 -> Saturation Dynamic/3

== system F16ASYM_Controlled_AoA/P controller + adaptive Crossed NN + AWU+Lim+scheduling   in AoA/Sigmoid  ==
  In : Inport
  Display : Display
  Fcn1 : Fcn  Commented=on  Expr=2.0 ./ (1.0 + exp(-u(4)*u(1:3)))-1
  MATLAB Function : MATLAB Function  TreatAsAtomicUnit=on
  a : Constant  Value=a
  Out : Outport
  wires:
  MATLAB Function/1(y) -> Display/1, Out/1
  In/1 -> MATLAB Function/1(u)
  a/1 -> MATLAB Function/2(a)

== system F16ASYM_Controlled_AoA/Primary Controller/P  + Crossed NN + AWU+Lim + hand-over ==
  note: Indicator correspond to 1
  note: Indicator correspond to 0
  A_w_z des : Inport
  AoA des (rad) : Inport  Port=2
  p des (rad/s) : Inport  Port=3
  beta des (rad) : Inport  Port=4
  Anti-windup A_w_z : Inport  Port=5
  Anti-windup AoA : Inport  Port=6
  Anti-windup beta : Inport  Port=7
  All measures : Inport  Port=8
  Anti-windup signals : Inport  Port=9
  A_w_z des1 : InportShadow
  Anti-windup A_w_z1 : InportShadow  Port=5
  Anti-windup AoA1 : InportShadow  Port=6
  Anti-windup beta1 : InportShadow  Port=7
  Anti-windup signals1 : InportShadow  Port=9
  AoA des (rad)1 : InportShadow  Port=2
  Bus Selector : BusSelector  OutputSignals=signal2.a,signal1.V_TAS (m/s)
  Gain2 : Gain  Gain=2
  Logical Operator : Logic  Operator=NOT  AllPortsSameDT=off  OutDataTypeStr=boolean
  Min TAS : Product  Inputs=**
  "P controller + adaptive Crossed NN + AWU+Lim    in ACC " : Subsystem  VariantObject=Adaptive Controller Crossed+AWU+Lim
  P controller + adaptive Crossed NN + AWU+Lim   in AoA : Subsystem  VariantObject=Adaptive Controller Crossed+AWU+Lim
  Relational Operator5 : RelationalOperator  OutDataTypeStr=boolean
  Scope : Scope
      settings: YMin=-2.75  YMax=0.25  SaveName=ScopeData32
  Scope1 : Scope  Commented=on
      settings: YMin=-2.75  YMax=0.25  SaveName=ScopeData33
  Switch : Switch  Commented=on  Threshold=0.5  InputSameDT=on
  Transition smoother : MATLAB Function  Commented=on  TreatAsAtomicUnit=on
  "Transitions Smotother " : Subsystem
  Transitions Smotother 1 : Subsystem  Commented=on
  Unit Delay : UnitDelay  Commented=on  SampleTime=-1
  beta des (rad)1 : InportShadow  Port=4
  p des (rad/s)1 : InportShadow  Port=3
  Angular acc des : Outport
  Control_in : Outport  Port=2
  wires:
  Anti-windup signals/1 -> P controller + adaptive Crossed NN + AWU+Lim   in AoA/9(Anti-windup signals)
  Anti-windup beta/1 -> P controller + adaptive Crossed NN + AWU+Lim   in AoA/7(Anti-windup beta)
  A_w_z des/1 -> P controller + adaptive Crossed NN + AWU+Lim   in AoA/1(A_w_z des)
  Anti-windup A_w_z/1 -> P controller + adaptive Crossed NN + AWU+Lim   in AoA/5(Anti-windup A_w_z)
  Anti-windup AoA/1 -> P controller + adaptive Crossed NN + AWU+Lim   in AoA/6(Anti-windup AoA)
  AoA des (rad)/1 -> P controller + adaptive Crossed NN + AWU+Lim   in AoA/2(AoA des (rad))
  beta des (rad)/1 -> P controller + adaptive Crossed NN + AWU+Lim   in AoA/4(beta des (rad))
  p des (rad/s)/1 -> P controller + adaptive Crossed NN + AWU+Lim   in AoA/3(p des (rad/s))
  A_w_z des1/1 -> "P controller + adaptive Crossed NN + AWU+Lim    in ACC "/1(A_w_z des)
  AoA des (rad)1/1 -> "P controller + adaptive Crossed NN + AWU+Lim    in ACC "/2(AoA des (rad))
  p des (rad/s)1/1 -> "P controller + adaptive Crossed NN + AWU+Lim    in ACC "/3(p des (rad/s))
  beta des (rad)1/1 -> "P controller + adaptive Crossed NN + AWU+Lim    in ACC "/4(beta des (rad))
  Anti-windup A_w_z1/1 -> "P controller + adaptive Crossed NN + AWU+Lim    in ACC "/5(Anti-windup A_w_z)
  Anti-windup AoA1/1 -> "P controller + adaptive Crossed NN + AWU+Lim    in ACC "/6(Anti-windup AoA)
  Anti-windup beta1/1 -> "P controller + adaptive Crossed NN + AWU+Lim    in ACC "/7(Anti-windup beta)
  All measures/1 -> "P controller + adaptive Crossed NN + AWU+Lim    in ACC "/8(All measures), Bus Selector/1, P controller + adaptive Crossed NN + AWU+Lim   in AoA/8(All measures)
  Anti-windup signals1/1 -> "P controller + adaptive Crossed NN + AWU+Lim    in ACC "/9(Anti-windup signals)
  [Min_Mach] -> Min TAS/1  "Min M"
  Bus Selector/1 -> Min TAS/2  "<a>"
  Min TAS/1 -> Gain2/1
  Gain2/1 -> Relational Operator5/1
  Bus Selector/2 -> Relational Operator5/2  "<V_TAS (m/s)>"
  "P controller + adaptive Crossed NN + AWU+Lim    in ACC "/1(Angular acc des) -> "Transitions Smotother "/3(From  ACC)
  P controller + adaptive Crossed NN + AWU+Lim   in AoA/1(Angular acc des) -> "Transitions Smotother "/1(From AoA)
  Relational Operator5/1 -> Logical Operator/1, Control_in/1, "Transitions Smotother "/2(Indicator), P controller + adaptive Crossed NN + AWU+Lim   in AoA/10(Active)
  Transition smoother/2(indicator_out) -> Unit Delay/1
  Unit Delay/1 -> Transition smoother/4(indicator_prev)
  "Transitions Smotother "/1(Ang accels comm) -> Angular acc des/1, Scope/1
  Switch/1 -> Scope1/1
  Logical Operator/1 -> "P controller + adaptive Crossed NN + AWU+Lim    in ACC "/10(Active)

== system F16ASYM_Controlled_AoA/Primary Controller/P controller ==
  A_w_z des : Inport
  AoA des (rad) : Inport  Port=2
  p des (rad/s) : Inport  Port=3
  beta des (rad) : Inport  Port=4
  Anti-windup A_w_z : Inport  Port=5
  Anti-windup AoA : Inport  Port=6
  Anti-windup beta : Inport  Port=7
  All measures : Inport  Port=8
  Anti-windup signals : Inport  Port=9
  Body Rates Controller : Subsystem
  Bus Creator2 : BusCreator
  Bus Selector3 : BusSelector  OutputSignals=signal1.SS meas (rad)
  Constant : Constant  Value=NaN
  Display : Display
  Display1 : Display
  Lat_dir Dyn Inversion: beta_dot->r_c : Subsystem
  Long Dyn Inversion: alpha_dot ->q : Subsystem
  Longitudinal Controller: AoA or A_w_z : Subsystem  Variant=on  OverrideUsingVariant=Controller of AoA
  Ref Model and P Controller : Adaptive_FaultTolerantControl/Ref Model and P Controller  tau=0.4  y_i=trim_state(9)  K_f=1  K_b=5
  Sum1 : Sum  Inputs=+-|
  Terminator : Terminator
  Terminator1 : Terminator
  Terminator2 : Terminator
  Angular acc des : Outport
  Control_in : Outport  Port=2
  wires:
  Anti-windup beta/1 -> Terminator1/1
  Ref Model and P Controller/5 -> Bus Creator2/4  "K_b_beta"
  Ref Model and P Controller/4 -> Sum1/2
  Sum1/1 -> Bus Creator2/3  "beta_err"
  Ref Model and P Controller/3 -> Bus Creator2/2, Sum1/1  "beta_sf"
  Ref Model and P Controller/2 -> Bus Creator2/1  "beta_sf_dot"
  Anti-windup signals/1 -> Terminator/1
  All measures/1 -> Longitudinal Controller: AoA or A_w_z/5(All meas), Long Dyn Inversion: alpha_dot ->q/2(All_meas), Bus Selector3/1, Lat_dir Dyn Inversion: beta_dot->r_c/2(All_meas), Body Rates Controller/4(All_meas)
  A_w_z des/1 -> Longitudinal Controller: AoA or A_w_z/1(A_w_z des)
  Anti-windup A_w_z/1 -> Longitudinal Controller: AoA or A_w_z/3(Anti-windup A_w_z)
  Anti-windup AoA/1 -> Longitudinal Controller: AoA or A_w_z/4(Anti-windup AoA)
  AoA des (rad)/1 -> Longitudinal Controller: AoA or A_w_z/2(AoA des (rad))
  Longitudinal Controller: AoA or A_w_z/3(alpha_dot_c) -> Display/1, Long Dyn Inversion: alpha_dot ->q/1(alpha_dot_c)
  beta des (rad)/1 -> Ref Model and P Controller/1
  Long Dyn Inversion: alpha_dot ->q/1(q_c) -> Body Rates Controller/2(q_ref), Display1/1
  p des (rad/s)/1 -> Body Rates Controller/1(p_ref)
  Ref Model and P Controller/1 -> Lat_dir Dyn Inversion: beta_dot->r_c/1(beta_dot_c)
  Bus Selector3/1 -> Ref Model and P Controller/2  "<SS meas (rad)>"
  Lat_dir Dyn Inversion: beta_dot->r_c/1(r_c) -> Body Rates Controller/3(r_ref)
  Bus Creator2/1 -> Terminator2/1  "beta_chanel vars"
  Body Rates Controller/1(Angular acc des (rad/s^2)) -> Angular acc des/1  "v_p+v_dot_ff"
  Constant/1 -> Control_in/1

== system F16ASYM_Controlled_AoA/Primary Controller/P controller + adaptive Crossed NN ==
  A_w_z des : Inport
  AoA des (rad) : Inport  Port=2
  p des (rad/s) : Inport  Port=3
  beta des (rad) : Inport  Port=4
  Anti-windup A_w_z : Inport  Port=5
  Anti-windup AoA : Inport  Port=6
  Anti-windup beta : Inport  Port=7
  All measures : Inport  Port=8
  Anti-windup signals : Inport  Port=9
  Body Rates Controller : Subsystem
  Bus Creator : BusCreator  Inputs=3
  Bus Creator1 : BusCreator  Inputs=3
  Bus Creator2 : BusCreator
  Bus Creator3 : BusCreator  Inputs=2
  Bus Selector3 : BusSelector  OutputSignals=signal1.SS meas (rad)
  Complete crossed On-line (adaptive) multi-layer NN : Subsystem  Variant=on  OverrideUsingVariant=NN on A_w_z
      mask Display:
      | image(imread('ANN.png'))
      | 
      | port_label('input', 1, 'v prev')
      | port_label('input', 2, 'All meas')
      | port_label('input', 3, 'NN vars')
      | 
      | port_label('output', 1, 'v_ad^')
  Display{,1..6} (7 alike) : Display
  Ground : Ground
  Lat_dir Dyn Inversion: beta_dot->r_c : Subsystem
  Long Dyn Inversion: alpha_dot ->q : Subsystem
  Longitudinal Controller: AoA or A_w_z : Subsystem  Variant=on  OverrideUsingVariant=Controller of A_w_z
  Memory : Memory  X0=[0,0,0]
  Ref Model and P Controller : Adaptive_FaultTolerantControl/Ref Model and P Controller  tau=0.45  y_i=trim_state(9)  K_f=1  K_b=5
  "Sigmoid " : Subsystem  mask{a=0.15}
      mask prompts: a "Sigmoid a param"
      mask TypeOptions a: a/Value
      mask Display:
      | x=-25:0.1:25;
      | 
      | y=(2.0 ./ (1.0 + exp(-a.*x))-1) ;
      | y2=zeros(size(x));
      | 
      | plot(x,y,x,y2);
      | 
      | text(-12,0.5, ['a= ',num2str(a)])
  Sum : Sum  Inputs=-+|
  Sum1 : Sum  Inputs=+-|
  Terminator : Terminator
  Terminator1 : Terminator
  Angular acc des : Outport
  Control_in : Outport  Port=2
  wires:
  Anti-windup signals/1 -> Terminator/1
  Ref Model and P Controller/1 -> Lat_dir Dyn Inversion: beta_dot->r_c/1(beta_dot_c), Display5/1
  Complete crossed On-line (adaptive) multi-layer NN/1(v_ad^) -> Display2/1, Sum/1  "v_ad^"
  "Sigmoid "/1(Out) -> Memory/1
  Anti-windup beta/1 -> Terminator1/1
  Bus Creator3/1 -> Bus Creator/3  "beta_r_chanel"
  Bus Creator2/1 -> Bus Creator3/2  "beta_chanel vars"
  Body Rates Controller/3(r_chanel vars) -> Bus Creator3/1  "r_chanel vars"
  Ref Model and P Controller/5 -> Bus Creator2/4  "K_b_beta"
  Ref Model and P Controller/4 -> Sum1/2
  Sum1/1 -> Bus Creator2/3  "beta_err"
  Ref Model and P Controller/3 -> Bus Creator2/2, Sum1/1  "beta_sf"
  Ref Model and P Controller/2 -> Bus Creator2/1  "beta_sf_dot"
  Bus Creator1/1 -> Bus Creator/1  "Long chanel"
  Longitudinal Controller: AoA or A_w_z/2(alpha_chanel vars) -> Bus Creator1/2  "alpha_chanel vars"
  Longitudinal Controller: AoA or A_w_z/1(A_chanel vars) -> Bus Creator1/1  "A_chanel vars"
  Body Rates Controller/1(q_chanel vars) -> Bus Creator1/3  "q_chanel_vars"
  Body Rates Controller/2(p_chanel vars) -> Bus Creator/2  "p_chanel_vars"
  Memory/1 -> Complete crossed On-line (adaptive) multi-layer NN/1(v_ad^ prev)
  Bus Creator/1 -> Complete crossed On-line (adaptive) multi-layer NN/3(NN variables)
  Body Rates Controller/4(Angular acc des (rad/s^2)) -> Sum/2, Display3/1  "v_p+v_dot_ff"
  All measures/1 -> Longitudinal Controller: AoA or A_w_z/5(All meas), Long Dyn Inversion: alpha_dot ->q/2(All_meas), Bus Selector3/1, Lat_dir Dyn Inversion: beta_dot->r_c/2(All_meas), Body Rates Controller/4(All_meas), Complete crossed On-line (adaptive) multi-layer NN/2(All_meas)
  Sum/1 -> Angular acc des/1, "Sigmoid "/1(In), Display4/1  "v"
  A_w_z des/1 -> Longitudinal Controller: AoA or A_w_z/1(A_w_z des)
  Anti-windup A_w_z/1 -> Longitudinal Controller: AoA or A_w_z/3(Anti-windup A_w_z)
  Anti-windup AoA/1 -> Longitudinal Controller: AoA or A_w_z/4(Anti-windup AoA)
  AoA des (rad)/1 -> Longitudinal Controller: AoA or A_w_z/2(AoA des (rad))
  Longitudinal Controller: AoA or A_w_z/3(alpha_dot_c) -> Display/1, Long Dyn Inversion: alpha_dot ->q/1(alpha_dot_c)
  beta des (rad)/1 -> Ref Model and P Controller/1
  Long Dyn Inversion: alpha_dot ->q/1(q_c) -> Body Rates Controller/2(q_ref), Display1/1
  p des (rad/s)/1 -> Body Rates Controller/1(p_ref)
  Bus Selector3/1 -> Ref Model and P Controller/2  "<SS meas (rad)>"
  Lat_dir Dyn Inversion: beta_dot->r_c/1(r_c) -> Body Rates Controller/3(r_ref), Display6/1
  Ground/1 -> Control_in/1
